simulink model "Accumulator"  (R2026a)
settings: Solver=VariableStepAuto
undefined symbols (not defined in the file): battery_builder_rtmsupport, gcbh
libraries: P5014s4pX10FINAL_lib x10, fl_lib x5, nesl_utility x4
settings Model: Creator=shlom  LastModifiedBy=shlom
settings SimscapeCC: SimscapeLogType=none

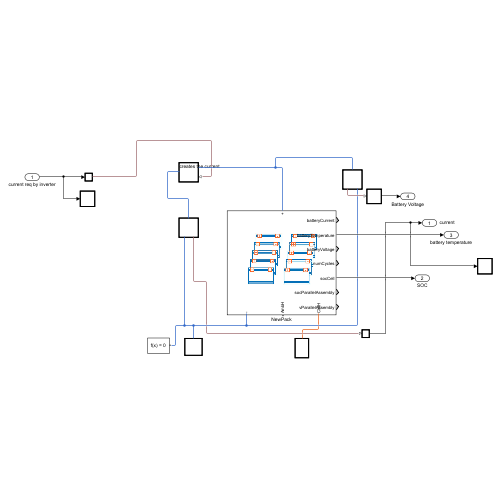
[thumbnail: Simulink's stored preview of the top-level diagram]
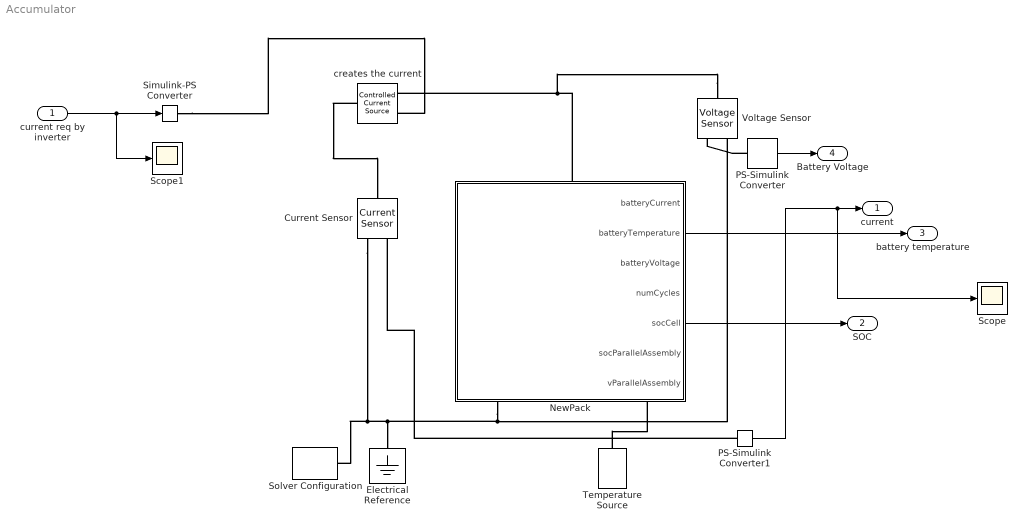
== system Accumulator ==
  current req by inverter : Inport
  Current Sensor : fl_lib/Electrical/Electrical Sensors/Current Sensor
  Electrical Reference : fl_lib/Electrical/Electrical Elements/Electrical Reference
  NewPack : Subsystem  LoadFcn=battery_builder_rtmsupport('loadfcn',gcbh);
      settings: CopyFcn=battery_builder_rtmsupport('copyfcn',gcbh);  PreCopyFcn=battery_builder_rtmsupport('precopyfcn',gcbh);  PreDeleteFcn=battery_builder_rtmsupport('predeletefcn',gcbh);  PortSchema="{\"entries\":[{\"content\":{\"sides\":[{\"content\":{\"connectorIds\":[\"LConn1\"]},\"type\":\"ConnectorPlacement.EquallySpacedRectSide\",\"uuid\":\"50a00692-8b3e-4b06-b9fd-9fe902dec650\"},{\"content\":{\"connectorIds\":[\"RConn1\",\"RConn2\",\"RConn3\"],\"side\":\"RIGHT\"},\"type\":\"ConnectorPlacement.EquallySpacedRectSide\",\"uuid\":\"1f4093e8-6f0b-4161-8c22-1274d739cfbf\"},{\"content\":{\"side\":\"TOP\"},\"type\":\"ConnectorPlacement.EquallySpacedRectSide\",\"uuid\":\"fed927fd-dc72-4186-a085-cad3a3e11086\"},{\"content\":{\"connectorIds\":[\"Out1\",\"Out2\",\"Out3\",\"Out4\",\"Out5\",\"Out6\",\"Out7\"],\"side\":\"BOTTOM\"},\"type\":\"ConnectorPlacement.EquallySpacedRectSide\",\"uuid\":\"8c9bd747-e275-4354-af9c-b2317d297e12\"}]},\"type\":\"ConnectorPlacement.EquallySpacedConnector\",\"uuid\":\"eabcc860-8705-4846-8283-0ad06230819d\"}],\"packageUris\":[\"http://schema.mathworks.com/mf0/Connector/R2020b\"],\"version\":\"1.0\"}"
      mask Display: image('$imagefile')
  PS-Simulink Converter : nesl_utility/PS-Simulink Converter  PhysicalDomain=network_engine_domain  SubClassName=ps_output  LeftPortType=input  RightPortType=output  PseudoPeriodic=off  Frequencies=[]  VectorFormat=inherit  Unit=inherit  AffineConversion=off
  PS-Simulink Converter1 : nesl_utility/PS-Simulink Converter  PhysicalDomain=network_engine_domain  SubClassName=ps_output  LeftPortType=input  RightPortType=output  PseudoPeriodic=off  Frequencies=[]  VectorFormat=inherit  Unit=inherit  AffineConversion=off
  Scope : Scope
      settings: ActiveDisplayYMinimum=-0.47222232529985531  ActiveDisplayYMaximum=0.055718666441431031
  Scope1 : Scope
      settings: ActiveDisplayYMinimum=-32.4079613538035  ActiveDisplayYMaximum=190.31249469621008
  Simulink-PS Converter : nesl_utility/Simulink-PS Converter  PhysicalDomain=network_engine_domain  SubClassName=ps_input  LeftPortType=input  RightPortType=output  PseudoPeriodic=off  Frequencies=[]  NoiseDistribution=none  NoiseParameters=[]  Unit=1  AffineConversion=off  FilteringAndDerivatives=provide  SimscapeFilterOrder=1  InputFilterTimeConstant=0.001  UdotUserProvided=0
  Solver Configuration : nesl_utility/Solver Configuration  PhysicalDomain=network_engine_domain  SubClassName=solver  LeftPortType=input  RightPortType=generic  Tones=[]  Harmonics=[]  SimulateNoise=off  Profile=off  UseLocalSampling=off  EnableSwitchedLinearOptims=on  FrequencyDomain=off  UseCCode=off  RelTol=0.001  AbsTol=0.001  MinStep=1e-09  ToWorkspace=off  RevertToSquareIcSolve=off  NumHomotopyIterations=100  PhasorMode=off  PhasorModeNumHarmonics=1  ConsistencySolver=NEWTON_XTOL_AFTER_FTOL  CanonicalOrdering=CANONICAL  OptimizeIntermediates=OPTIMIZED  IndexReductionMethod=DerivativeReplacement  DoDC=off  ResidualTolerance=1e-09  ConsistencyTolSource=GLOBAL  ConsistencyAbsTol=0.001  ConsistencyRelTol=0.001  ConsistencyTolFactor=0.001  UseLocalSolver=off  LocalSolverChoice=NE_BACKWARD_EULER_ADVANCER  ResolveIndetEquations=on  FunctionEvalNumThread=1  LocalSolverSampleTime=0.001  DoFixedCost=off  MaxNonlinIter=3  MaxModeIter=2  ComputeImpulses=off  ImpulseIterations=2  LinearAlgebra=auto  LinearAlgebraNumThread=0  EquationFormulation=NE_TIME_EF  DelaysMemoryBudget=1024  AutomaticFiltering=on  FilteringTimeConstant=0.001  PartitionStorageMethod=AS_NEEDED  PartitionMemoryBudget=1024  PartitionMethod=ROBUST  MultibodyUseLocalSolver=off  MultibodyLocalSolverChoice=ODE1  MultibodyLocalSolverSampleTime=0.001
  Temperature Source : fl_lib/Thermal/Thermal Sources/Temperature Source  temperature=330 K
  Voltage Sensor : fl_lib/Electrical/Electrical Sensors/Voltage Sensor
  creates the current : fl_lib/Electrical/Electrical Sources/Controlled Current Source
  current : Outport
  SOC : Outport  Port=2
  battery temperature : Outport  Port=3
  Battery Voltage : Outport  Port=4
  wires:
  NewPack/5(socCell) -> SOC/1
  NewPack/2(batteryTemperature) -> battery temperature/1
  current req by inverter/1 -> Scope1/1, Simulink-PS Converter/1
  PS-Simulink Converter/1 -> Battery Voltage/1
  PS-Simulink Converter1/1 -> Scope/1, current/1
  connections:
  Voltage Sensor/LConn1 -- NewPack/LConn1 -- creates the current/RConn2
  Simulink-PS Converter/RConn1 -- creates the current/RConn1
  NewPack/RConn1 -- Voltage Sensor/RConn2 -- Electrical Reference/LConn1 -- Current Sensor/RConn2 -- Solver Configuration/RConn1
  PS-Simulink Converter/LConn1 -- Voltage Sensor/RConn1
  creates the current/LConn1 -- Current Sensor/LConn1
  PS-Simulink Converter1/LConn1 -- Current Sensor/RConn1
  Temperature Source/LConn1 -- NewPack/RConn3

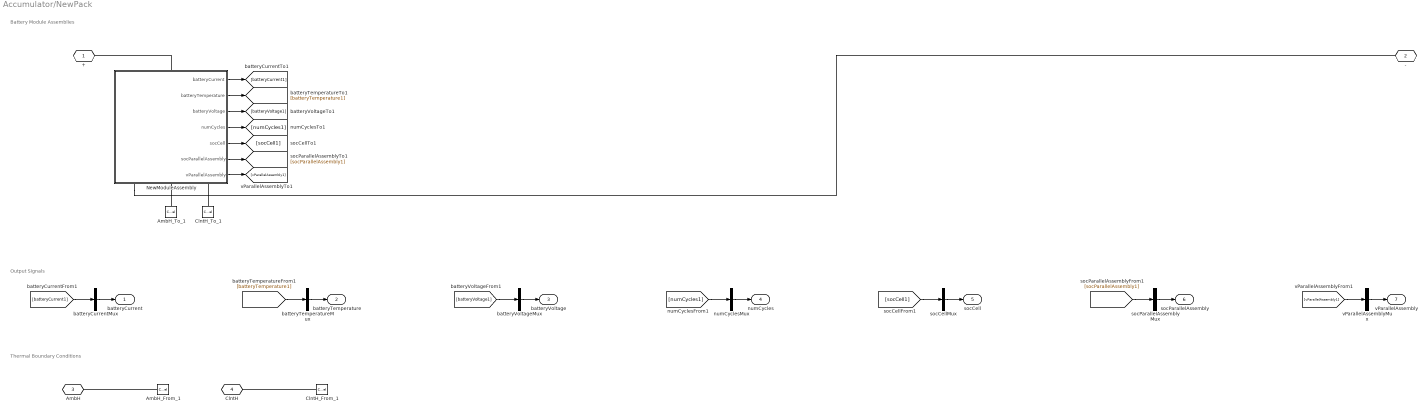
== system Accumulator/NewPack ==
  note: Thermal Boundary Conditions
  note: Output Signals
  note: Battery Module Assemblies
  AmbH_From_1 : ConnectionLabel  Label=ambH_1
  AmbH_To_1 : ConnectionLabel  Label=ambH_1
  ClntH_From_1 : ConnectionLabel  Label=clntH_1
  ClntH_To_1 : ConnectionLabel  Label=clntH_1
  NewModuleAssembly : Subsystem  LoadFcn=battery_builder_rtmsupport('loadfcn',gcbh);
      settings: CopyFcn=battery_builder_rtmsupport('copyfcn',gcbh);  PreCopyFcn=battery_builder_rtmsupport('precopyfcn',gcbh);  PreDeleteFcn=battery_builder_rtmsupport('predeletefcn',gcbh);  PortSchema="{\"entries\":[{\"content\":{\"sides\":[{\"content\":{\"connectorIds\":[\"LConn1\"]},\"type\":\"ConnectorPlacement.EquallySpacedRectSide\",\"uuid\":\"50a00692-8b3e-4b06-b9fd-9fe902dec650\"},{\"content\":{\"connectorIds\":[\"RConn1\",\"RConn2\",\"RConn3\"],\"side\":\"RIGHT\"},\"type\":\"ConnectorPlacement.EquallySpacedRectSide\",\"uuid\":\"1f4093e8-6f0b-4161-8c22-1274d739cfbf\"},{\"content\":{\"side\":\"TOP\"},\"type\":\"ConnectorPlacement.EquallySpacedRectSide\",\"uuid\":\"fed927fd-dc72-4186-a085-cad3a3e11086\"},{\"content\":{\"connectorIds\":[\"Out1\",\"Out2\",\"Out3\",\"Out4\",\"Out5\",\"Out6\",\"Out7\"],\"side\":\"BOTTOM\"},\"type\":\"ConnectorPlacement.EquallySpacedRectSide\",\"uuid\":\"cf6fc4bd-b2c0-45cd-8752-1112b57d821c\"}]},\"type\":\"ConnectorPlacement.EquallySpacedConnector\",\"uuid\":\"eabcc860-8705-4846-8283-0ad06230819d\"}],\"packageUris\":[\"http://schema.mathworks.com/mf0/Connector/R2020b\"],\"version\":\"1.0\"}"
      mask Display: image('$imagefile')
  batteryCurrentMux : Mux  Inputs=1
  batteryTemperatureMux : Mux  Inputs=1
  batteryVoltageMux : Mux  Inputs=1
  numCyclesMux : Mux  Inputs=1
  socCellMux : Mux  Inputs=1
  socParallelAssemblyMux : Mux  Inputs=1
  vParallelAssemblyMux : Mux  Inputs=1
  + : PMIOPort  Side=Left
  - : PMIOPort  Port=2  Side=Right
  AmbH : PMIOPort  Port=3  Side=Right  ConnectionType=Connection: foundation.thermal.thermal
  ClntH : PMIOPort  Port=4  Side=Right  ConnectionType=Connection: foundation.thermal.thermal
  batteryCurrent : Outport
  batteryTemperature : Outport  Port=2
  batteryVoltage : Outport  Port=3
  numCycles : Outport  Port=4
  socCell : Outport  Port=5
  socParallelAssembly : Outport  Port=6
  vParallelAssembly : Outport  Port=7
  wires:
  [vParallelAssembly1] -> vParallelAssemblyMux/1
  vParallelAssemblyMux/1 -> vParallelAssembly/1
  NewModuleAssembly/7(vParallelAssembly) -> [vParallelAssembly1]
  [socParallelAssembly1] -> socParallelAssemblyMux/1
  socParallelAssemblyMux/1 -> socParallelAssembly/1
  NewModuleAssembly/6(socParallelAssembly) -> [socParallelAssembly1]
  [socCell1] -> socCellMux/1
  socCellMux/1 -> socCell/1
  NewModuleAssembly/5(socCell) -> [socCell1]
  [numCycles1] -> numCyclesMux/1
  numCyclesMux/1 -> numCycles/1
  NewModuleAssembly/4(numCycles) -> [numCycles1]
  [batteryVoltage1] -> batteryVoltageMux/1
  batteryVoltageMux/1 -> batteryVoltage/1
  NewModuleAssembly/3(batteryVoltage) -> [batteryVoltage1]
  [batteryTemperature1] -> batteryTemperatureMux/1
  batteryTemperatureMux/1 -> batteryTemperature/1
  NewModuleAssembly/2(batteryTemperature) -> [batteryTemperature1]
  [batteryCurrent1] -> batteryCurrentMux/1
  batteryCurrentMux/1 -> batteryCurrent/1
  NewModuleAssembly/1(batteryCurrent) -> [batteryCurrent1]
  connections:
  ClntH_From_1/LConn1 -- ClntH/RConn1
  ClntH_To_1/LConn1 -- NewModuleAssembly/RConn3
  AmbH_From_1/LConn1 -- AmbH/RConn1
  AmbH_To_1/LConn1 -- NewModuleAssembly/RConn2
  NewModuleAssembly/RConn1 -- -/RConn1
  NewModuleAssembly/LConn1 -- +/RConn1

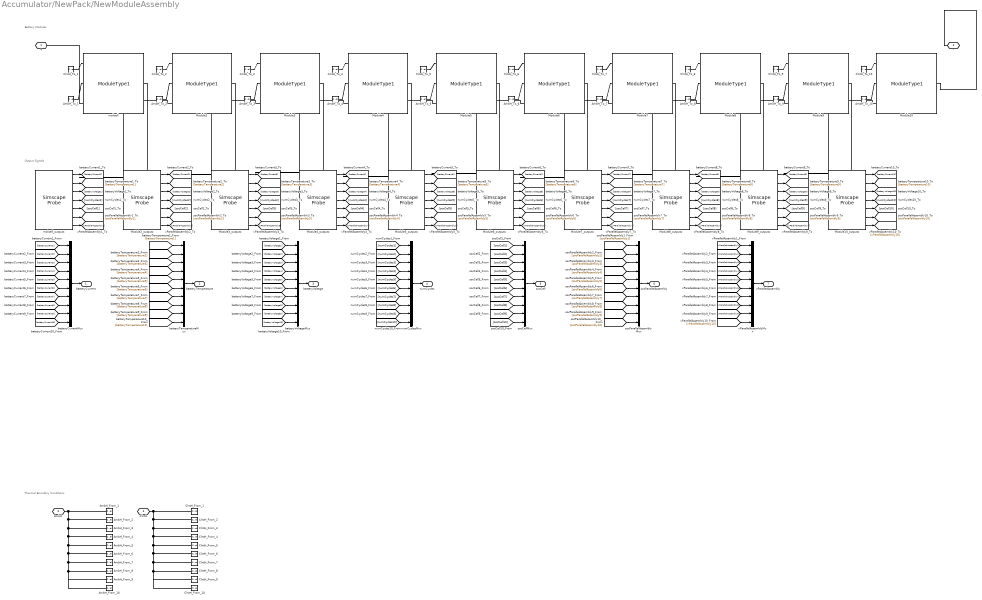
== system Accumulator/NewPack/NewModuleAssembly ==
  note: Battery Modules
  note: Output Signals
  note: Thermal Boundary Conditions
  AmbH_From_1 : ConnectionLabel  Label=ambH_1
  AmbH_From_10 : ConnectionLabel  Label=ambH_10
  AmbH_From_2 : ConnectionLabel  Label=ambH_2
  AmbH_From_3 : ConnectionLabel  Label=ambH_3
  AmbH_From_4 : ConnectionLabel  Label=ambH_4
  AmbH_From_5 : ConnectionLabel  Label=ambH_5
  AmbH_From_6 : ConnectionLabel  Label=ambH_6
  AmbH_From_7 : ConnectionLabel  Label=ambH_7
  AmbH_From_8 : ConnectionLabel  Label=ambH_8
  AmbH_From_9 : ConnectionLabel  Label=ambH_9
  AmbH_To_1 : ConnectionLabel  Label=ambH_1
  AmbH_To_10 : ConnectionLabel  Label=ambH_10
  AmbH_To_2 : ConnectionLabel  Label=ambH_2
  AmbH_To_3 : ConnectionLabel  Label=ambH_3
  AmbH_To_4 : ConnectionLabel  Label=ambH_4
  AmbH_To_5 : ConnectionLabel  Label=ambH_5
  AmbH_To_6 : ConnectionLabel  Label=ambH_6
  AmbH_To_7 : ConnectionLabel  Label=ambH_7
  AmbH_To_8 : ConnectionLabel  Label=ambH_8
  AmbH_To_9 : ConnectionLabel  Label=ambH_9
  ClntH_From_1 : ConnectionLabel  Label=clntH_1
  ClntH_From_10 : ConnectionLabel  Label=clntH_10
  ClntH_From_2 : ConnectionLabel  Label=clntH_2
  ClntH_From_3 : ConnectionLabel  Label=clntH_3
  ClntH_From_4 : ConnectionLabel  Label=clntH_4
  ClntH_From_5 : ConnectionLabel  Label=clntH_5
  ClntH_From_6 : ConnectionLabel  Label=clntH_6
  ClntH_From_7 : ConnectionLabel  Label=clntH_7
  ClntH_From_8 : ConnectionLabel  Label=clntH_8
  ClntH_From_9 : ConnectionLabel  Label=clntH_9
  ClntH_To_1 : ConnectionLabel  Label=clntH_1
  ClntH_To_10 : ConnectionLabel  Label=clntH_10
  ClntH_To_2 : ConnectionLabel  Label=clntH_2
  ClntH_To_3 : ConnectionLabel  Label=clntH_3
  ClntH_To_4 : ConnectionLabel  Label=clntH_4
  ClntH_To_5 : ConnectionLabel  Label=clntH_5
  ClntH_To_6 : ConnectionLabel  Label=clntH_6
  ClntH_To_7 : ConnectionLabel  Label=clntH_7
  ClntH_To_8 : ConnectionLabel  Label=clntH_8
  ClntH_To_9 : ConnectionLabel  Label=clntH_9
  Module10 : P5014s4pX10FINAL_lib/Modules/ModuleType1  BatteryCapacityCell=NewModuleAssembly.Module10.BatteryCapacityCell A*hr  ExtrapolationMethodCell=simscape.enum.extrapolation.linear  SOCBreakpointsCell=NewModuleAssembly.Module10.SOCBreakpointsCell  TemperatureBreakpointsCell=NewModuleAssembly.Module10.TemperatureBreakpointsCell degC  OpenCircuitVoltageThermalCell=NewModuleAssembly.Module10.OpenCircuitVoltageThermalCell V  VoltageRangeCell=NewModuleAssembly.Module10.VoltageRangeCell V  ResistanceSOCBreakpointsCell=NewModuleAssembly.Module10.ResistanceSOCBreakpointsCell  ResistanceTemperatureBreakpointsCell=NewModuleAssembly.Module10.ResistanceTemperatureBreakpointsCell degC  R0ThermalCell=NewModuleAssembly.Module10.R0ThermalCell Ohm  BatteryThermalMassCell=NewModuleAssembly.Module10.BatteryThermalMassCell J/K  CoolantResistance=NewModuleAssembly.Module10.CoolantResistance K/W  AmbientResistance=NewModuleAssembly.Module10.AmbientResistance K/W  socCell_specify=off  socCell_priority=High  socCell=1  socCell_nominal_specify=off  socCell_nominal_value=1  socCell_nominal_unit=1  batteryVoltage_specify=off  batteryVoltage_priority=None  batteryVoltage=0 V  batteryVoltage_nominal_specify=off  batteryVoltage_nominal_value=1  batteryVoltage_nominal_unit=V  batteryCurrent_specify=off  batteryCurrent_priority=None  batteryCurrent=0 A  batteryCurrent_nominal_specify=off  batteryCurrent_nominal_value=1  batteryCurrent_nominal_unit=A  numCycles_specify=off  numCycles_priority=High  numCycles=0  numCycles_nominal_specify=off  numCycles_nominal_value=1  numCycles_nominal_unit=1  batteryTemperature_specify=off  batteryTemperature_priority=High  batteryTemperature=298.15 K  batteryTemperature_nominal_specify=off  batteryTemperature_nominal_value=1  batteryTemperature_nominal_unit=K  vParallelAssembly_specify=off  vParallelAssembly_priority=None  vParallelAssembly=repmat(0, 14, 1) V  vParallelAssembly_nominal_specify=off  vParallelAssembly_nominal_value=1  vParallelAssembly_nominal_unit=V  socParallelAssembly_specify=off  socParallelAssembly_priority=None  socParallelAssembly=repmat(1, 14, 1)  socParallelAssembly_nominal_specify=off  socParallelAssembly_nominal_value=1  socParallelAssembly_nominal_unit=1
  Module10_outputs : SimscapeProbe  BoundBlock=5584  Variables="{\"batteryCurrent\":{\"Probing\":\"ON\"},\"batteryTemperature\":{\"Probing\":\"ON\"},\"batteryVoltage\":{\"Probing\":\"ON\"},\"numCycles\":{\"Probing\":\"ON\"},\"socCell\":{\"Probing\":\"ON\"},\"socParallelAssembly\":{\"Probing\":\"ON\"},\"vParallelAssembly\":{\"Probing\":\"ON\"}}"
  Module2 : P5014s4pX10FINAL_lib/Modules/ModuleType1  BatteryCapacityCell=NewModuleAssembly.Module2.BatteryCapacityCell A*hr  ExtrapolationMethodCell=simscape.enum.extrapolation.linear  SOCBreakpointsCell=NewModuleAssembly.Module2.SOCBreakpointsCell  TemperatureBreakpointsCell=NewModuleAssembly.Module2.TemperatureBreakpointsCell degC  OpenCircuitVoltageThermalCell=NewModuleAssembly.Module2.OpenCircuitVoltageThermalCell V  VoltageRangeCell=NewModuleAssembly.Module2.VoltageRangeCell V  ResistanceSOCBreakpointsCell=NewModuleAssembly.Module2.ResistanceSOCBreakpointsCell  ResistanceTemperatureBreakpointsCell=NewModuleAssembly.Module2.ResistanceTemperatureBreakpointsCell degC  R0ThermalCell=NewModuleAssembly.Module2.R0ThermalCell Ohm  BatteryThermalMassCell=NewModuleAssembly.Module2.BatteryThermalMassCell J/K  CoolantResistance=NewModuleAssembly.Module2.CoolantResistance K/W  AmbientResistance=NewModuleAssembly.Module2.AmbientResistance K/W  socCell_specify=off  socCell_priority=High  socCell=1  socCell_nominal_specify=off  socCell_nominal_value=1  socCell_nominal_unit=1  batteryVoltage_specify=off  batteryVoltage_priority=None  batteryVoltage=0 V  batteryVoltage_nominal_specify=off  batteryVoltage_nominal_value=1  batteryVoltage_nominal_unit=V  batteryCurrent_specify=off  batteryCurrent_priority=None  batteryCurrent=0 A  batteryCurrent_nominal_specify=off  batteryCurrent_nominal_value=1  batteryCurrent_nominal_unit=A  numCycles_specify=off  numCycles_priority=High  numCycles=0  numCycles_nominal_specify=off  numCycles_nominal_value=1  numCycles_nominal_unit=1  batteryTemperature_specify=off  batteryTemperature_priority=High  batteryTemperature=298.15 K  batteryTemperature_nominal_specify=off  batteryTemperature_nominal_value=1  batteryTemperature_nominal_unit=K  vParallelAssembly_specify=off  vParallelAssembly_priority=None  vParallelAssembly=repmat(0, 14, 1) V  vParallelAssembly_nominal_specify=off  vParallelAssembly_nominal_value=1  vParallelAssembly_nominal_unit=V  socParallelAssembly_specify=off  socParallelAssembly_priority=None  socParallelAssembly=repmat(1, 14, 1)  socParallelAssembly_nominal_specify=off  socParallelAssembly_nominal_value=1  socParallelAssembly_nominal_unit=1
  Module2_outputs : SimscapeProbe  BoundBlock=5586  Variables="{\"batteryCurrent\":{\"Probing\":\"ON\"},\"batteryTemperature\":{\"Probing\":\"ON\"},\"batteryVoltage\":{\"Probing\":\"ON\"},\"numCycles\":{\"Probing\":\"ON\"},\"socCell\":{\"Probing\":\"ON\"},\"socParallelAssembly\":{\"Probing\":\"ON\"},\"vParallelAssembly\":{\"Probing\":\"ON\"}}"
  Module3 : P5014s4pX10FINAL_lib/Modules/ModuleType1  BatteryCapacityCell=NewModuleAssembly.Module3.BatteryCapacityCell A*hr  ExtrapolationMethodCell=simscape.enum.extrapolation.linear  SOCBreakpointsCell=NewModuleAssembly.Module3.SOCBreakpointsCell  TemperatureBreakpointsCell=NewModuleAssembly.Module3.TemperatureBreakpointsCell degC  OpenCircuitVoltageThermalCell=NewModuleAssembly.Module3.OpenCircuitVoltageThermalCell V  VoltageRangeCell=NewModuleAssembly.Module3.VoltageRangeCell V  ResistanceSOCBreakpointsCell=NewModuleAssembly.Module3.ResistanceSOCBreakpointsCell  ResistanceTemperatureBreakpointsCell=NewModuleAssembly.Module3.ResistanceTemperatureBreakpointsCell degC  R0ThermalCell=NewModuleAssembly.Module3.R0ThermalCell Ohm  BatteryThermalMassCell=NewModuleAssembly.Module3.BatteryThermalMassCell J/K  CoolantResistance=NewModuleAssembly.Module3.CoolantResistance K/W  AmbientResistance=NewModuleAssembly.Module3.AmbientResistance K/W  socCell_specify=off  socCell_priority=High  socCell=1  socCell_nominal_specify=off  socCell_nominal_value=1  socCell_nominal_unit=1  batteryVoltage_specify=off  batteryVoltage_priority=None  batteryVoltage=0 V  batteryVoltage_nominal_specify=off  batteryVoltage_nominal_value=1  batteryVoltage_nominal_unit=V  batteryCurrent_specify=off  batteryCurrent_priority=None  batteryCurrent=0 A  batteryCurrent_nominal_specify=off  batteryCurrent_nominal_value=1  batteryCurrent_nominal_unit=A  numCycles_specify=off  numCycles_priority=High  numCycles=0  numCycles_nominal_specify=off  numCycles_nominal_value=1  numCycles_nominal_unit=1  batteryTemperature_specify=off  batteryTemperature_priority=High  batteryTemperature=298.15 K  batteryTemperature_nominal_specify=off  batteryTemperature_nominal_value=1  batteryTemperature_nominal_unit=K  vParallelAssembly_specify=off  vParallelAssembly_priority=None  vParallelAssembly=repmat(0, 14, 1) V  vParallelAssembly_nominal_specify=off  vParallelAssembly_nominal_value=1  vParallelAssembly_nominal_unit=V  socParallelAssembly_specify=off  socParallelAssembly_priority=None  socParallelAssembly=repmat(1, 14, 1)  socParallelAssembly_nominal_specify=off  socParallelAssembly_nominal_value=1  socParallelAssembly_nominal_unit=1
  Module3_outputs : SimscapeProbe  BoundBlock=5588  Variables="{\"batteryCurrent\":{\"Probing\":\"ON\"},\"batteryTemperature\":{\"Probing\":\"ON\"},\"batteryVoltage\":{\"Probing\":\"ON\"},\"numCycles\":{\"Probing\":\"ON\"},\"socCell\":{\"Probing\":\"ON\"},\"socParallelAssembly\":{\"Probing\":\"ON\"},\"vParallelAssembly\":{\"Probing\":\"ON\"}}"
  Module4 : P5014s4pX10FINAL_lib/Modules/ModuleType1  BatteryCapacityCell=NewModuleAssembly.Module4.BatteryCapacityCell A*hr  ExtrapolationMethodCell=simscape.enum.extrapolation.linear  SOCBreakpointsCell=NewModuleAssembly.Module4.SOCBreakpointsCell  TemperatureBreakpointsCell=NewModuleAssembly.Module4.TemperatureBreakpointsCell degC  OpenCircuitVoltageThermalCell=NewModuleAssembly.Module4.OpenCircuitVoltageThermalCell V  VoltageRangeCell=NewModuleAssembly.Module4.VoltageRangeCell V  ResistanceSOCBreakpointsCell=NewModuleAssembly.Module4.ResistanceSOCBreakpointsCell  ResistanceTemperatureBreakpointsCell=NewModuleAssembly.Module4.ResistanceTemperatureBreakpointsCell degC  R0ThermalCell=NewModuleAssembly.Module4.R0ThermalCell Ohm  BatteryThermalMassCell=NewModuleAssembly.Module4.BatteryThermalMassCell J/K  CoolantResistance=NewModuleAssembly.Module4.CoolantResistance K/W  AmbientResistance=NewModuleAssembly.Module4.AmbientResistance K/W  socCell_specify=off  socCell_priority=High  socCell=1  socCell_nominal_specify=off  socCell_nominal_value=1  socCell_nominal_unit=1  batteryVoltage_specify=off  batteryVoltage_priority=None  batteryVoltage=0 V  batteryVoltage_nominal_specify=off  batteryVoltage_nominal_value=1  batteryVoltage_nominal_unit=V  batteryCurrent_specify=off  batteryCurrent_priority=None  batteryCurrent=0 A  batteryCurrent_nominal_specify=off  batteryCurrent_nominal_value=1  batteryCurrent_nominal_unit=A  numCycles_specify=off  numCycles_priority=High  numCycles=0  numCycles_nominal_specify=off  numCycles_nominal_value=1  numCycles_nominal_unit=1  batteryTemperature_specify=off  batteryTemperature_priority=High  batteryTemperature=298.15 K  batteryTemperature_nominal_specify=off  batteryTemperature_nominal_value=1  batteryTemperature_nominal_unit=K  vParallelAssembly_specify=off  vParallelAssembly_priority=None  vParallelAssembly=repmat(0, 14, 1) V  vParallelAssembly_nominal_specify=off  vParallelAssembly_nominal_value=1  vParallelAssembly_nominal_unit=V  socParallelAssembly_specify=off  socParallelAssembly_priority=None  socParallelAssembly=repmat(1, 14, 1)  socParallelAssembly_nominal_specify=off  socParallelAssembly_nominal_value=1  socParallelAssembly_nominal_unit=1
  Module4_outputs : SimscapeProbe  BoundBlock=5590  Variables="{\"batteryCurrent\":{\"Probing\":\"ON\"},\"batteryTemperature\":{\"Probing\":\"ON\"},\"batteryVoltage\":{\"Probing\":\"ON\"},\"numCycles\":{\"Probing\":\"ON\"},\"socCell\":{\"Probing\":\"ON\"},\"socParallelAssembly\":{\"Probing\":\"ON\"},\"vParallelAssembly\":{\"Probing\":\"ON\"}}"
  Module5 : P5014s4pX10FINAL_lib/Modules/ModuleType1  BatteryCapacityCell=NewModuleAssembly.Module5.BatteryCapacityCell A*hr  ExtrapolationMethodCell=simscape.enum.extrapolation.linear  SOCBreakpointsCell=NewModuleAssembly.Module5.SOCBreakpointsCell  TemperatureBreakpointsCell=NewModuleAssembly.Module5.TemperatureBreakpointsCell degC  OpenCircuitVoltageThermalCell=NewModuleAssembly.Module5.OpenCircuitVoltageThermalCell V  VoltageRangeCell=NewModuleAssembly.Module5.VoltageRangeCell V  ResistanceSOCBreakpointsCell=NewModuleAssembly.Module5.ResistanceSOCBreakpointsCell  ResistanceTemperatureBreakpointsCell=NewModuleAssembly.Module5.ResistanceTemperatureBreakpointsCell degC  R0ThermalCell=NewModuleAssembly.Module5.R0ThermalCell Ohm  BatteryThermalMassCell=NewModuleAssembly.Module5.BatteryThermalMassCell J/K  CoolantResistance=NewModuleAssembly.Module5.CoolantResistance K/W  AmbientResistance=NewModuleAssembly.Module5.AmbientResistance K/W  socCell_specify=off  socCell_priority=High  socCell=1  socCell_nominal_specify=off  socCell_nominal_value=1  socCell_nominal_unit=1  batteryVoltage_specify=off  batteryVoltage_priority=None  batteryVoltage=0 V  batteryVoltage_nominal_specify=off  batteryVoltage_nominal_value=1  batteryVoltage_nominal_unit=V  batteryCurrent_specify=off  batteryCurrent_priority=None  batteryCurrent=0 A  batteryCurrent_nominal_specify=off  batteryCurrent_nominal_value=1  batteryCurrent_nominal_unit=A  numCycles_specify=off  numCycles_priority=High  numCycles=0  numCycles_nominal_specify=off  numCycles_nominal_value=1  numCycles_nominal_unit=1  batteryTemperature_specify=off  batteryTemperature_priority=High  batteryTemperature=298.15 K  batteryTemperature_nominal_specify=off  batteryTemperature_nominal_value=1  batteryTemperature_nominal_unit=K  vParallelAssembly_specify=off  vParallelAssembly_priority=None  vParallelAssembly=repmat(0, 14, 1) V  vParallelAssembly_nominal_specify=off  vParallelAssembly_nominal_value=1  vParallelAssembly_nominal_unit=V  socParallelAssembly_specify=off  socParallelAssembly_priority=None  socParallelAssembly=repmat(1, 14, 1)  socParallelAssembly_nominal_specify=off  socParallelAssembly_nominal_value=1  socParallelAssembly_nominal_unit=1
  Module5_outputs : SimscapeProbe  BoundBlock=5592  Variables="{\"batteryCurrent\":{\"Probing\":\"ON\"},\"batteryTemperature\":{\"Probing\":\"ON\"},\"batteryVoltage\":{\"Probing\":\"ON\"},\"numCycles\":{\"Probing\":\"ON\"},\"socCell\":{\"Probing\":\"ON\"},\"socParallelAssembly\":{\"Probing\":\"ON\"},\"vParallelAssembly\":{\"Probing\":\"ON\"}}"
  Module6 : P5014s4pX10FINAL_lib/Modules/ModuleType1  BatteryCapacityCell=NewModuleAssembly.Module6.BatteryCapacityCell A*hr  ExtrapolationMethodCell=simscape.enum.extrapolation.linear  SOCBreakpointsCell=NewModuleAssembly.Module6.SOCBreakpointsCell  TemperatureBreakpointsCell=NewModuleAssembly.Module6.TemperatureBreakpointsCell degC  OpenCircuitVoltageThermalCell=NewModuleAssembly.Module6.OpenCircuitVoltageThermalCell V  VoltageRangeCell=NewModuleAssembly.Module6.VoltageRangeCell V  ResistanceSOCBreakpointsCell=NewModuleAssembly.Module6.ResistanceSOCBreakpointsCell  ResistanceTemperatureBreakpointsCell=NewModuleAssembly.Module6.ResistanceTemperatureBreakpointsCell degC  R0ThermalCell=NewModuleAssembly.Module6.R0ThermalCell Ohm  BatteryThermalMassCell=NewModuleAssembly.Module6.BatteryThermalMassCell J/K  CoolantResistance=NewModuleAssembly.Module6.CoolantResistance K/W  AmbientResistance=NewModuleAssembly.Module6.AmbientResistance K/W  socCell_specify=off  socCell_priority=High  socCell=1  socCell_nominal_specify=off  socCell_nominal_value=1  socCell_nominal_unit=1  batteryVoltage_specify=off  batteryVoltage_priority=None  batteryVoltage=0 V  batteryVoltage_nominal_specify=off  batteryVoltage_nominal_value=1  batteryVoltage_nominal_unit=V  batteryCurrent_specify=off  batteryCurrent_priority=None  batteryCurrent=0 A  batteryCurrent_nominal_specify=off  batteryCurrent_nominal_value=1  batteryCurrent_nominal_unit=A  numCycles_specify=off  numCycles_priority=High  numCycles=0  numCycles_nominal_specify=off  numCycles_nominal_value=1  numCycles_nominal_unit=1  batteryTemperature_specify=off  batteryTemperature_priority=High  batteryTemperature=298.15 K  batteryTemperature_nominal_specify=off  batteryTemperature_nominal_value=1  batteryTemperature_nominal_unit=K  vParallelAssembly_specify=off  vParallelAssembly_priority=None  vParallelAssembly=repmat(0, 14, 1) V  vParallelAssembly_nominal_specify=off  vParallelAssembly_nominal_value=1  vParallelAssembly_nominal_unit=V  socParallelAssembly_specify=off  socParallelAssembly_priority=None  socParallelAssembly=repmat(1, 14, 1)  socParallelAssembly_nominal_specify=off  socParallelAssembly_nominal_value=1  socParallelAssembly_nominal_unit=1
  Module6_outputs : SimscapeProbe  BoundBlock=5594  Variables="{\"batteryCurrent\":{\"Probing\":\"ON\"},\"batteryTemperature\":{\"Probing\":\"ON\"},\"batteryVoltage\":{\"Probing\":\"ON\"},\"numCycles\":{\"Probing\":\"ON\"},\"socCell\":{\"Probing\":\"ON\"},\"socParallelAssembly\":{\"Probing\":\"ON\"},\"vParallelAssembly\":{\"Probing\":\"ON\"}}"
  Module7 : P5014s4pX10FINAL_lib/Modules/ModuleType1  BatteryCapacityCell=NewModuleAssembly.Module7.BatteryCapacityCell A*hr  ExtrapolationMethodCell=simscape.enum.extrapolation.linear  SOCBreakpointsCell=NewModuleAssembly.Module7.SOCBreakpointsCell  TemperatureBreakpointsCell=NewModuleAssembly.Module7.TemperatureBreakpointsCell degC  OpenCircuitVoltageThermalCell=NewModuleAssembly.Module7.OpenCircuitVoltageThermalCell V  VoltageRangeCell=NewModuleAssembly.Module7.VoltageRangeCell V  ResistanceSOCBreakpointsCell=NewModuleAssembly.Module7.ResistanceSOCBreakpointsCell  ResistanceTemperatureBreakpointsCell=NewModuleAssembly.Module7.ResistanceTemperatureBreakpointsCell degC  R0ThermalCell=NewModuleAssembly.Module7.R0ThermalCell Ohm  BatteryThermalMassCell=NewModuleAssembly.Module7.BatteryThermalMassCell J/K  CoolantResistance=NewModuleAssembly.Module7.CoolantResistance K/W  AmbientResistance=NewModuleAssembly.Module7.AmbientResistance K/W  socCell_specify=off  socCell_priority=High  socCell=1  socCell_nominal_specify=off  socCell_nominal_value=1  socCell_nominal_unit=1  batteryVoltage_specify=off  batteryVoltage_priority=None  batteryVoltage=0 V  batteryVoltage_nominal_specify=off  batteryVoltage_nominal_value=1  batteryVoltage_nominal_unit=V  batteryCurrent_specify=off  batteryCurrent_priority=None  batteryCurrent=0 A  batteryCurrent_nominal_specify=off  batteryCurrent_nominal_value=1  batteryCurrent_nominal_unit=A  numCycles_specify=off  numCycles_priority=High  numCycles=0  numCycles_nominal_specify=off  numCycles_nominal_value=1  numCycles_nominal_unit=1  batteryTemperature_specify=off  batteryTemperature_priority=High  batteryTemperature=298.15 K  batteryTemperature_nominal_specify=off  batteryTemperature_nominal_value=1  batteryTemperature_nominal_unit=K  vParallelAssembly_specify=off  vParallelAssembly_priority=None  vParallelAssembly=repmat(0, 14, 1) V  vParallelAssembly_nominal_specify=off  vParallelAssembly_nominal_value=1  vParallelAssembly_nominal_unit=V  socParallelAssembly_specify=off  socParallelAssembly_priority=None  socParallelAssembly=repmat(1, 14, 1)  socParallelAssembly_nominal_specify=off  socParallelAssembly_nominal_value=1  socParallelAssembly_nominal_unit=1
  Module7_outputs : SimscapeProbe  BoundBlock=5596  Variables="{\"batteryCurrent\":{\"Probing\":\"ON\"},\"batteryTemperature\":{\"Probing\":\"ON\"},\"batteryVoltage\":{\"Probing\":\"ON\"},\"numCycles\":{\"Probing\":\"ON\"},\"socCell\":{\"Probing\":\"ON\"},\"socParallelAssembly\":{\"Probing\":\"ON\"},\"vParallelAssembly\":{\"Probing\":\"ON\"}}"
  Module8 : P5014s4pX10FINAL_lib/Modules/ModuleType1  BatteryCapacityCell=NewModuleAssembly.Module8.BatteryCapacityCell A*hr  ExtrapolationMethodCell=simscape.enum.extrapolation.linear  SOCBreakpointsCell=NewModuleAssembly.Module8.SOCBreakpointsCell  TemperatureBreakpointsCell=NewModuleAssembly.Module8.TemperatureBreakpointsCell degC  OpenCircuitVoltageThermalCell=NewModuleAssembly.Module8.OpenCircuitVoltageThermalCell V  VoltageRangeCell=NewModuleAssembly.Module8.VoltageRangeCell V  ResistanceSOCBreakpointsCell=NewModuleAssembly.Module8.ResistanceSOCBreakpointsCell  ResistanceTemperatureBreakpointsCell=NewModuleAssembly.Module8.ResistanceTemperatureBreakpointsCell degC  R0ThermalCell=NewModuleAssembly.Module8.R0ThermalCell Ohm  BatteryThermalMassCell=NewModuleAssembly.Module8.BatteryThermalMassCell J/K  CoolantResistance=NewModuleAssembly.Module8.CoolantResistance K/W  AmbientResistance=NewModuleAssembly.Module8.AmbientResistance K/W  socCell_specify=off  socCell_priority=High  socCell=1  socCell_nominal_specify=off  socCell_nominal_value=1  socCell_nominal_unit=1  batteryVoltage_specify=off  batteryVoltage_priority=None  batteryVoltage=0 V  batteryVoltage_nominal_specify=off  batteryVoltage_nominal_value=1  batteryVoltage_nominal_unit=V  batteryCurrent_specify=off  batteryCurrent_priority=None  batteryCurrent=0 A  batteryCurrent_nominal_specify=off  batteryCurrent_nominal_value=1  batteryCurrent_nominal_unit=A  numCycles_specify=off  numCycles_priority=High  numCycles=0  numCycles_nominal_specify=off  numCycles_nominal_value=1  numCycles_nominal_unit=1  batteryTemperature_specify=off  batteryTemperature_priority=High  batteryTemperature=298.15 K  batteryTemperature_nominal_specify=off  batteryTemperature_nominal_value=1  batteryTemperature_nominal_unit=K  vParallelAssembly_specify=off  vParallelAssembly_priority=None  vParallelAssembly=repmat(0, 14, 1) V  vParallelAssembly_nominal_specify=off  vParallelAssembly_nominal_value=1  vParallelAssembly_nominal_unit=V  socParallelAssembly_specify=off  socParallelAssembly_priority=None  socParallelAssembly=repmat(1, 14, 1)  socParallelAssembly_nominal_specify=off  socParallelAssembly_nominal_value=1  socParallelAssembly_nominal_unit=1
  Module8_outputs : SimscapeProbe  BoundBlock=5598  Variables="{\"batteryCurrent\":{\"Probing\":\"ON\"},\"batteryTemperature\":{\"Probing\":\"ON\"},\"batteryVoltage\":{\"Probing\":\"ON\"},\"numCycles\":{\"Probing\":\"ON\"},\"socCell\":{\"Probing\":\"ON\"},\"socParallelAssembly\":{\"Probing\":\"ON\"},\"vParallelAssembly\":{\"Probing\":\"ON\"}}"
  Module9 : P5014s4pX10FINAL_lib/Modules/ModuleType1  BatteryCapacityCell=NewModuleAssembly.Module9.BatteryCapacityCell A*hr  ExtrapolationMethodCell=simscape.enum.extrapolation.linear  SOCBreakpointsCell=NewModuleAssembly.Module9.SOCBreakpointsCell  TemperatureBreakpointsCell=NewModuleAssembly.Module9.TemperatureBreakpointsCell degC  OpenCircuitVoltageThermalCell=NewModuleAssembly.Module9.OpenCircuitVoltageThermalCell V  VoltageRangeCell=NewModuleAssembly.Module9.VoltageRangeCell V  ResistanceSOCBreakpointsCell=NewModuleAssembly.Module9.ResistanceSOCBreakpointsCell  ResistanceTemperatureBreakpointsCell=NewModuleAssembly.Module9.ResistanceTemperatureBreakpointsCell degC  R0ThermalCell=NewModuleAssembly.Module9.R0ThermalCell Ohm  BatteryThermalMassCell=NewModuleAssembly.Module9.BatteryThermalMassCell J/K  CoolantResistance=NewModuleAssembly.Module9.CoolantResistance K/W  AmbientResistance=NewModuleAssembly.Module9.AmbientResistance K/W  socCell_specify=off  socCell_priority=High  socCell=1  socCell_nominal_specify=off  socCell_nominal_value=1  socCell_nominal_unit=1  batteryVoltage_specify=off  batteryVoltage_priority=None  batteryVoltage=0 V  batteryVoltage_nominal_specify=off  batteryVoltage_nominal_value=1  batteryVoltage_nominal_unit=V  batteryCurrent_specify=off  batteryCurrent_priority=None  batteryCurrent=0 A  batteryCurrent_nominal_specify=off  batteryCurrent_nominal_value=1  batteryCurrent_nominal_unit=A  numCycles_specify=off  numCycles_priority=High  numCycles=0  numCycles_nominal_specify=off  numCycles_nominal_value=1  numCycles_nominal_unit=1  batteryTemperature_specify=off  batteryTemperature_priority=High  batteryTemperature=298.15 K  batteryTemperature_nominal_specify=off  batteryTemperature_nominal_value=1  batteryTemperature_nominal_unit=K  vParallelAssembly_specify=off  vParallelAssembly_priority=None  vParallelAssembly=repmat(0, 14, 1) V  vParallelAssembly_nominal_specify=off  vParallelAssembly_nominal_value=1  vParallelAssembly_nominal_unit=V  socParallelAssembly_specify=off  socParallelAssembly_priority=None  socParallelAssembly=repmat(1, 14, 1)  socParallelAssembly_nominal_specify=off  socParallelAssembly_nominal_value=1  socParallelAssembly_nominal_unit=1
  Module9_outputs : SimscapeProbe  BoundBlock=5600  Variables="{\"batteryCurrent\":{\"Probing\":\"ON\"},\"batteryTemperature\":{\"Probing\":\"ON\"},\"batteryVoltage\":{\"Probing\":\"ON\"},\"numCycles\":{\"Probing\":\"ON\"},\"socCell\":{\"Probing\":\"ON\"},\"socParallelAssembly\":{\"Probing\":\"ON\"},\"vParallelAssembly\":{\"Probing\":\"ON\"}}"
  batteryCurrentMux : Mux  Inputs=10
  batteryTemperatureMux : Mux  Inputs=10
  batteryVoltageMux : Mux  Inputs=10
  molicell : P5014s4pX10FINAL_lib/Modules/ModuleType1  BatteryCapacityCell=NewModuleAssembly.molicell.BatteryCapacityCell A*hr  ExtrapolationMethodCell=simscape.enum.extrapolation.linear  SOCBreakpointsCell=NewModuleAssembly.molicell.SOCBreakpointsCell  TemperatureBreakpointsCell=NewModuleAssembly.molicell.TemperatureBreakpointsCell degC  OpenCircuitVoltageThermalCell=NewModuleAssembly.molicell.OpenCircuitVoltageThermalCell V  VoltageRangeCell=NewModuleAssembly.molicell.VoltageRangeCell V  ResistanceSOCBreakpointsCell=NewModuleAssembly.molicell.ResistanceSOCBreakpointsCell  ResistanceTemperatureBreakpointsCell=NewModuleAssembly.molicell.ResistanceTemperatureBreakpointsCell degC  R0ThermalCell=NewModuleAssembly.molicell.R0ThermalCell Ohm  BatteryThermalMassCell=NewModuleAssembly.molicell.BatteryThermalMassCell J/K  CoolantResistance=NewModuleAssembly.molicell.CoolantResistance K/W  AmbientResistance=NewModuleAssembly.molicell.AmbientResistance K/W  socCell_specify=off  socCell_priority=High  socCell=1  socCell_nominal_specify=off  socCell_nominal_value=1  socCell_nominal_unit=1  batteryVoltage_specify=off  batteryVoltage_priority=None  batteryVoltage=0 V  batteryVoltage_nominal_specify=off  batteryVoltage_nominal_value=1  batteryVoltage_nominal_unit=V  batteryCurrent_specify=off  batteryCurrent_priority=None  batteryCurrent=0 A  batteryCurrent_nominal_specify=off  batteryCurrent_nominal_value=1  batteryCurrent_nominal_unit=A  numCycles_specify=off  numCycles_priority=High  numCycles=0  numCycles_nominal_specify=off  numCycles_nominal_value=1  numCycles_nominal_unit=1  batteryTemperature_specify=off  batteryTemperature_priority=High  batteryTemperature=298.15 K  batteryTemperature_nominal_specify=off  batteryTemperature_nominal_value=1  batteryTemperature_nominal_unit=K  vParallelAssembly_specify=off  vParallelAssembly_priority=None  vParallelAssembly=repmat(0, 14, 1) V  vParallelAssembly_nominal_specify=off  vParallelAssembly_nominal_value=1  vParallelAssembly_nominal_unit=V  socParallelAssembly_specify=off  socParallelAssembly_priority=None  socParallelAssembly=repmat(1, 14, 1)  socParallelAssembly_nominal_specify=off  socParallelAssembly_nominal_value=1  socParallelAssembly_nominal_unit=1
  molicell_outputs : SimscapeProbe  BoundBlock=5665  Variables="{\"batteryCurrent\":{\"Probing\":\"ON\"},\"batteryTemperature\":{\"Probing\":\"ON\"},\"batteryVoltage\":{\"Probing\":\"ON\"},\"numCycles\":{\"Probing\":\"ON\"},\"socCell\":{\"Probing\":\"ON\"},\"socParallelAssembly\":{\"Probing\":\"ON\"},\"vParallelAssembly\":{\"Probing\":\"ON\"}}"
  numCyclesMux : Mux  Inputs=10
  socCellMux : Mux  Inputs=10
  socParallelAssemblyMux : Mux  Inputs=10
  vParallelAssemblyMux : Mux  Inputs=10
  + : PMIOPort  Side=Left
  - : PMIOPort  Port=2  Side=Right
  AmbH : PMIOPort  Port=3  Side=Right  ConnectionType=Connection: foundation.thermal.thermal
  ClntH : PMIOPort  Port=4  Side=Right  ConnectionType=Connection: foundation.thermal.thermal
  batteryCurrent : Outport
  batteryTemperature : Outport  Port=2
  batteryVoltage : Outport  Port=3
  numCycles : Outport  Port=4
  socCell : Outport  Port=5
  socParallelAssembly : Outport  Port=6
  vParallelAssembly : Outport  Port=7
  wires:
  molicell_outputs/1 -> [batteryCurrent1]
  batteryCurrentMux/1 -> batteryCurrent/1
  [batteryCurrent1] -> batteryCurrentMux/1
  molicell_outputs/2 -> [batteryTemperature1]
  batteryTemperatureMux/1 -> batteryTemperature/1
  [batteryTemperature1] -> batteryTemperatureMux/1
  molicell_outputs/3 -> [batteryVoltage1]
  batteryVoltageMux/1 -> batteryVoltage/1
  [batteryVoltage1] -> batteryVoltageMux/1
  molicell_outputs/4 -> [numCycles1]
  numCyclesMux/1 -> numCycles/1
  [numCycles1] -> numCyclesMux/1
  molicell_outputs/5 -> [socCell1]
  socCellMux/1 -> socCell/1
  [socCell1] -> socCellMux/1
  molicell_outputs/6 -> [socParallelAssembly1]
  socParallelAssemblyMux/1 -> socParallelAssembly/1
  [socParallelAssembly1] -> socParallelAssemblyMux/1
  molicell_outputs/7 -> [vParallelAssembly1]
  vParallelAssemblyMux/1 -> vParallelAssembly/1
  [vParallelAssembly1] -> vParallelAssemblyMux/1
  Module2_outputs/1 -> [batteryCurrent2]
  [batteryCurrent2] -> batteryCurrentMux/2
  Module2_outputs/2 -> [batteryTemperature2]
  [batteryTemperature2] -> batteryTemperatureMux/2
  Module2_outputs/3 -> [batteryVoltage2]
  [batteryVoltage2] -> batteryVoltageMux/2
  Module2_outputs/4 -> [numCycles2]
  [numCycles2] -> numCyclesMux/2
  Module2_outputs/5 -> [socCell2]
  [socCell2] -> socCellMux/2
  Module2_outputs/6 -> [socParallelAssembly2]
  [socParallelAssembly2] -> socParallelAssemblyMux/2
  Module2_outputs/7 -> [vParallelAssembly2]
  [vParallelAssembly2] -> vParallelAssemblyMux/2
  Module3_outputs/1 -> [batteryCurrent3]
  [batteryCurrent3] -> batteryCurrentMux/3
  Module3_outputs/2 -> [batteryTemperature3]
  [batteryTemperature3] -> batteryTemperatureMux/3
  Module3_outputs/3 -> [batteryVoltage3]
  [batteryVoltage3] -> batteryVoltageMux/3
  Module3_outputs/4 -> [numCycles3]
  [numCycles3] -> numCyclesMux/3
  Module3_outputs/5 -> [socCell3]
  [socCell3] -> socCellMux/3
  Module3_outputs/6 -> [socParallelAssembly3]
  [socParallelAssembly3] -> socParallelAssemblyMux/3
  Module3_outputs/7 -> [vParallelAssembly3]
  [vParallelAssembly3] -> vParallelAssemblyMux/3
  Module4_outputs/1 -> [batteryCurrent4]
  [batteryCurrent4] -> batteryCurrentMux/4
  Module4_outputs/2 -> [batteryTemperature4]
  [batteryTemperature4] -> batteryTemperatureMux/4
  Module4_outputs/3 -> [batteryVoltage4]
  [batteryVoltage4] -> batteryVoltageMux/4
  Module4_outputs/4 -> [numCycles4]
  [numCycles4] -> numCyclesMux/4
  Module4_outputs/5 -> [socCell4]
  [socCell4] -> socCellMux/4
  Module4_outputs/6 -> [socParallelAssembly4]
  [socParallelAssembly4] -> socParallelAssemblyMux/4
  Module4_outputs/7 -> [vParallelAssembly4]
  [vParallelAssembly4] -> vParallelAssemblyMux/4
  Module5_outputs/1 -> [batteryCurrent5]
  [batteryCurrent5] -> batteryCurrentMux/5
  Module5_outputs/2 -> [batteryTemperature5]
  [batteryTemperature5] -> batteryTemperatureMux/5
  Module5_outputs/3 -> [batteryVoltage5]
  [batteryVoltage5] -> batteryVoltageMux/5
  Module5_outputs/4 -> [numCycles5]
  [numCycles5] -> numCyclesMux/5
  Module5_outputs/5 -> [socCell5]
  [socCell5] -> socCellMux/5
  Module5_outputs/6 -> [socParallelAssembly5]
  [socParallelAssembly5] -> socParallelAssemblyMux/5
  Module5_outputs/7 -> [vParallelAssembly5]
  [vParallelAssembly5] -> vParallelAssemblyMux/5
  Module6_outputs/1 -> [batteryCurrent6]
  [batteryCurrent6] -> batteryCurrentMux/6
  Module6_outputs/2 -> [batteryTemperature6]
  [batteryTemperature6] -> batteryTemperatureMux/6
  Module6_outputs/3 -> [batteryVoltage6]
  [batteryVoltage6] -> batteryVoltageMux/6
  Module6_outputs/4 -> [numCycles6]
  [numCycles6] -> numCyclesMux/6
  Module6_outputs/5 -> [socCell6]
  [socCell6] -> socCellMux/6
  Module6_outputs/6 -> [socParallelAssembly6]
  [socParallelAssembly6] -> socParallelAssemblyMux/6
  Module6_outputs/7 -> [vParallelAssembly6]
  [vParallelAssembly6] -> vParallelAssemblyMux/6
  Module7_outputs/1 -> [batteryCurrent7]
  [batteryCurrent7] -> batteryCurrentMux/7
  Module7_outputs/2 -> [batteryTemperature7]
  [batteryTemperature7] -> batteryTemperatureMux/7
  Module7_outputs/3 -> [batteryVoltage7]
  [batteryVoltage7] -> batteryVoltageMux/7
  Module7_outputs/4 -> [numCycles7]
  [numCycles7] -> numCyclesMux/7
  Module7_outputs/5 -> [socCell7]
  [socCell7] -> socCellMux/7
  Module7_outputs/6 -> [socParallelAssembly7]
  [socParallelAssembly7] -> socParallelAssemblyMux/7
  Module7_outputs/7 -> [vParallelAssembly7]
  [vParallelAssembly7] -> vParallelAssemblyMux/7
  Module8_outputs/1 -> [batteryCurrent8]
  [batteryCurrent8] -> batteryCurrentMux/8
  Module8_outputs/2 -> [batteryTemperature8]
  [batteryTemperature8] -> batteryTemperatureMux/8
  Module8_outputs/3 -> [batteryVoltage8]
  [batteryVoltage8] -> batteryVoltageMux/8
  Module8_outputs/4 -> [numCycles8]
  [numCycles8] -> numCyclesMux/8
  Module8_outputs/5 -> [socCell8]
  [socCell8] -> socCellMux/8
  Module8_outputs/6 -> [socParallelAssembly8]
  [socParallelAssembly8] -> socParallelAssemblyMux/8
  Module8_outputs/7 -> [vParallelAssembly8]
  [vParallelAssembly8] -> vParallelAssemblyMux/8
  Module9_outputs/1 -> [batteryCurrent9]
  [batteryCurrent9] -> batteryCurrentMux/9
  Module9_outputs/2 -> [batteryTemperature9]
  [batteryTemperature9] -> batteryTemperatureMux/9
  Module9_outputs/3 -> [batteryVoltage9]
  [batteryVoltage9] -> batteryVoltageMux/9
  Module9_outputs/4 -> [numCycles9]
  [numCycles9] -> numCyclesMux/9
  Module9_outputs/5 -> [socCell9]
  [socCell9] -> socCellMux/9
  Module9_outputs/6 -> [socParallelAssembly9]
  [socParallelAssembly9] -> socParallelAssemblyMux/9
  Module9_outputs/7 -> [vParallelAssembly9]
  [vParallelAssembly9] -> vParallelAssemblyMux/9
  Module10_outputs/1 -> [batteryCurrent10]
  [batteryCurrent10] -> batteryCurrentMux/10
  Module10_outputs/2 -> [batteryTemperature10]
  [batteryTemperature10] -> batteryTemperatureMux/10
  Module10_outputs/3 -> [batteryVoltage10]
  [batteryVoltage10] -> batteryVoltageMux/10
  Module10_outputs/4 -> [numCycles10]
  [numCycles10] -> numCyclesMux/10
  Module10_outputs/5 -> [socCell10]
  [socCell10] -> socCellMux/10
  Module10_outputs/6 -> [socParallelAssembly10]
  [socParallelAssembly10] -> socParallelAssemblyMux/10
  Module10_outputs/7 -> [vParallelAssembly10]
  [vParallelAssembly10] -> vParallelAssemblyMux/10
  connections:
  Module2/LConn3 -- molicell/RConn1
  Module3/LConn3 -- Module2/RConn1
  Module4/LConn3 -- Module3/RConn1
  Module5/LConn3 -- Module4/RConn1
  Module6/LConn3 -- Module5/RConn1
  Module7/LConn3 -- Module6/RConn1
  Module8/LConn3 -- Module7/RConn1
  Module9/LConn3 -- Module8/RConn1
  Module10/LConn3 -- Module9/RConn1
  molicell/LConn3 -- +/RConn1
  Module10/RConn1 -- -/RConn1
  AmbH_To_1/LConn1 -- molicell/LConn2
  AmbH_From_9/LConn1 -- AmbH_From_10/LConn1 -- AmbH_From_8/LConn1 -- AmbH_From_7/LConn1 -- AmbH_From_6/LConn1 -- AmbH_From_5/LConn1 -- AmbH_From_4/LConn1 -- AmbH_From_3/LConn1 -- AmbH_From_2/LConn1 -- AmbH_From_1/LConn1 -- AmbH/RConn1
  AmbH_To_2/LConn1 -- Module2/LConn2
  AmbH_To_3/LConn1 -- Module3/LConn2
  AmbH_To_4/LConn1 -- Module4/LConn2
  AmbH_To_5/LConn1 -- Module5/LConn2
  AmbH_To_6/LConn1 -- Module6/LConn2
  AmbH_To_7/LConn1 -- Module7/LConn2
  AmbH_To_8/LConn1 -- Module8/LConn2
  AmbH_To_9/LConn1 -- Module9/LConn2
  AmbH_To_10/LConn1 -- Module10/LConn2
  ClntH_To_1/LConn1 -- molicell/LConn1
  ClntH_From_9/LConn1 -- ClntH_From_10/LConn1 -- ClntH_From_8/LConn1 -- ClntH_From_7/LConn1 -- ClntH_From_6/LConn1 -- ClntH_From_5/LConn1 -- ClntH_From_4/LConn1 -- ClntH_From_3/LConn1 -- ClntH_From_2/LConn1 -- ClntH_From_1/LConn1 -- ClntH/RConn1
  ClntH_To_2/LConn1 -- Module2/LConn1
  ClntH_To_3/LConn1 -- Module3/LConn1
  ClntH_To_4/LConn1 -- Module4/LConn1
  ClntH_To_5/LConn1 -- Module5/LConn1
  ClntH_To_6/LConn1 -- Module6/LConn1
  ClntH_To_7/LConn1 -- Module7/LConn1
  ClntH_To_8/LConn1 -- Module8/LConn1
  ClntH_To_9/LConn1 -- Module9/LConn1
  ClntH_To_10/LConn1 -- Module10/LConn1
